simulink model "pro82"  (Simulink 7.4)
settings: Solver=ode45  StartTime=0.0  StopTime=10.0  RelTol=1e-3
undefined symbols (not defined in the file or in its folder): magnitude
libraries: commchan3 x20, commfilt2 x8, dspstat3 x4, dspindex x2, commdigbbndpm3 x2, dspinverses x2, commrandsrc2 x1, commsink2 x1
settings Model: Creator=tjh  LastModifiedBy=tjh

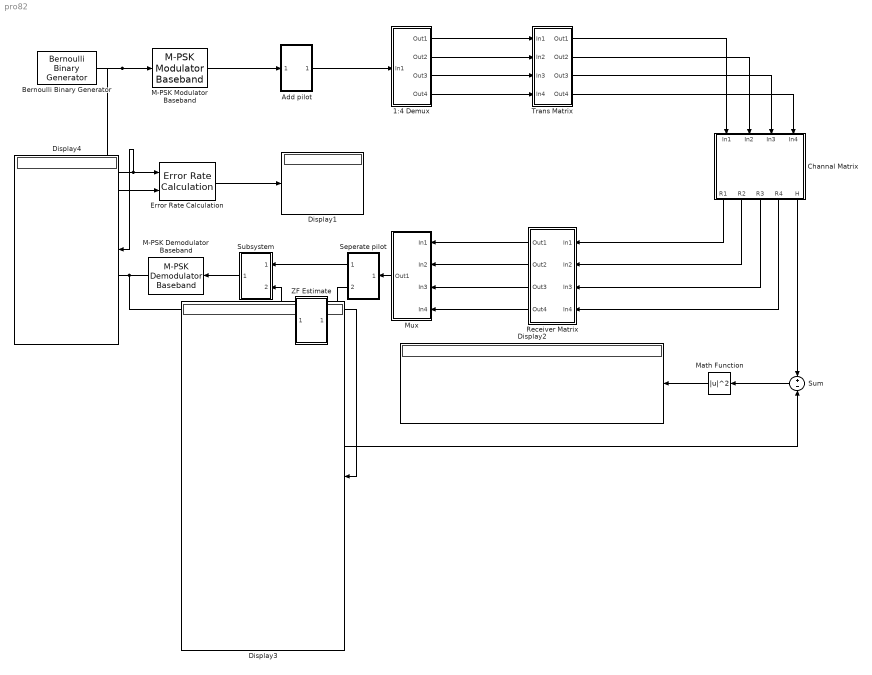
== system pro82 ==
  1:4 Demux : Subsystem
  Add pilot : Subsystem
  Bernoulli Binary Generator : commrandsrc2/Bernoulli Binary Generator  DialogController=commDDGCreate  DialogControllerArgs=DataTag0  SystemSampleTime=-1  P=0.5  seed=61  Ts=1e-4/(4*4*96)  frameBased=on  sampPerFrame=4*4*96  orient=off  outDataType=boolean
  Channal Matrix : Subsystem
  Display{1..4} (4 alike) : Display
  Error Rate Calculation : commsink2/Error Rate Calculation  N=21  st_delay=0  cp_mode=Entire frame  subframe=[]  PMode=Port  WsName=ErrorVec  RsMode2=off  stop=off  numErr=100  maxBits=1e6
  M-PSK Demodulator Baseband : commdigbbndpm3/M-PSK Demodulator Baseband  DialogController=commDDGCreate  DialogControllerArgs=DataTag5  M=16  Ph=pi/16  Dec=Gray  Mapping=[0:7]  OutType=Bit  DecType=Hard decision  VarSource=Dialog  Variance=1  outDtype1=boolean  outDtype2=Inherit via internal rule  derotateFactorWordLen=16
  M-PSK Modulator Baseband : commdigbbndpm3/M-PSK Modulator Baseband  DialogController=commDDGCreate  DialogControllerArgs=DataTag6  M=16  InType=Bit  Enc=Gray  Mapping=[0:7]  Ph=pi/16  outDtype=double  outWordLen=16  outUDDataType=sfix(16)  outFracLenMode=Best precision  outFracLen=15
  Math Function : Math  Operator=magnitude^2  OutDataType=fixdt(1, 16)  OutScaling=2^0  SaturateOnIntegerOverflow=on
  Mux : Subsystem
  Receiver Matrix : Subsystem
  Seperate pilot : Subsystem
  Subsystem : Subsystem
  Sum : Sum  Inputs=+-  OutDataType=fixdt(1, 16)  OutScaling=2^0
  Trans Matrix : Subsystem
  ZF Estimate : Subsystem
  wires:
  Bernoulli Binary Generator/1 -> M-PSK Modulator Baseband/1, Error Rate Calculation/1, Display4/1
  M-PSK Modulator Baseband/1 -> Add pilot/1(In1)
  Add pilot/1(Out1) -> 1:4 Demux/1(In1)
  1:4 Demux/1(Out1) -> Trans Matrix/1(In1)
  1:4 Demux/2(Out2) -> Trans Matrix/2(In2)
  1:4 Demux/3(Out3) -> Trans Matrix/3(In3)
  1:4 Demux/4(Out4) -> Trans Matrix/4(In4)
  Trans Matrix/1(Out1) -> Channal Matrix/1(In1)
  Trans Matrix/3(Out3) -> Channal Matrix/3(In3)
  Channal Matrix/1(R1) -> Receiver Matrix/1(In1)
  Trans Matrix/2(Out2) -> Channal Matrix/2(In2)
  Trans Matrix/4(Out4) -> Channal Matrix/4(In4)
  Channal Matrix/2(R2) -> Receiver Matrix/2(In2)
  Channal Matrix/3(R3) -> Receiver Matrix/3(In3)
  Channal Matrix/4(R4) -> Receiver Matrix/4(In4)
  Receiver Matrix/1(Out1) -> Mux/1(In1)
  Receiver Matrix/2(Out2) -> Mux/2(In2)
  Receiver Matrix/3(Out3) -> Mux/3(In3)
  Receiver Matrix/4(Out4) -> Mux/4(In4)
  Mux/1(Out1) -> Seperate pilot/1(In1)
  Seperate pilot/2(Out2) -> ZF Estimate/1(In1)
  ZF Estimate/1(Out1) -> Subsystem/2(In2), Sum/2
  Seperate pilot/1(Out1) -> Subsystem/1(In1)
  Subsystem/1(Out1) -> M-PSK Demodulator Baseband/1
  M-PSK Demodulator Baseband/1 -> Error Rate Calculation/2, Display3/1
  Error Rate Calculation/1 -> Display1/1
  Channal Matrix/5(H) -> Sum/1
  Sum/1 -> Math Function/1
  Math Function/1 -> Display2/1

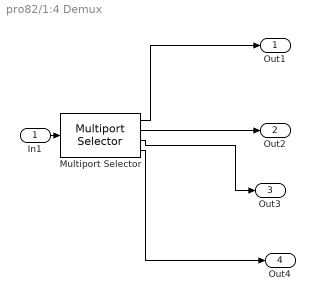
== system pro82/1:4 Demux ==
  In1 : Inport
  Multiport Selector : dspindex/Multiport Selector  rowsOrCols=Rows  idxCellArray={ 1, 2, 3, 4 }  idxErrMode=Clip Index
  Out1 : Outport
  Out2 : Outport  Port=2
  Out3 : Outport  Port=3
  Out4 : Outport  Port=4
  wires:
  Multiport Selector/1 -> Out1/1
  Multiport Selector/2 -> Out2/1
  In1/1 -> Multiport Selector/1
  Multiport Selector/3 -> Out3/1
  Multiport Selector/4 -> Out4/1

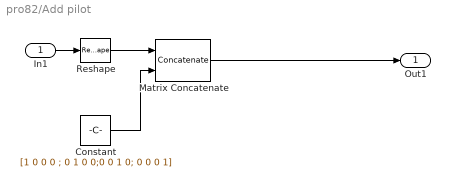
== system pro82/Add pilot ==
  In1 : Inport
  Constant : Constant  Value=[1 0 0 0 ; 0 1 0 0;0 0 1 0; 0 0 0 1]  OutDataType=fixdt(1, 16)  OutScaling=2^0  SampleTime=1e-4
  Matrix Concatenate : Concatenate  Mode=Multidimensional array  ConcatenateDimension=2
  Reshape : Reshape  OutputDimensionality=Customize  OutputDimensions=[4,96]
  Out1 : Outport
  wires:
  Reshape/1 -> Matrix Concatenate/1
  Constant/1 -> Matrix Concatenate/2
  In1/1 -> Reshape/1
  Matrix Concatenate/1 -> Out1/1

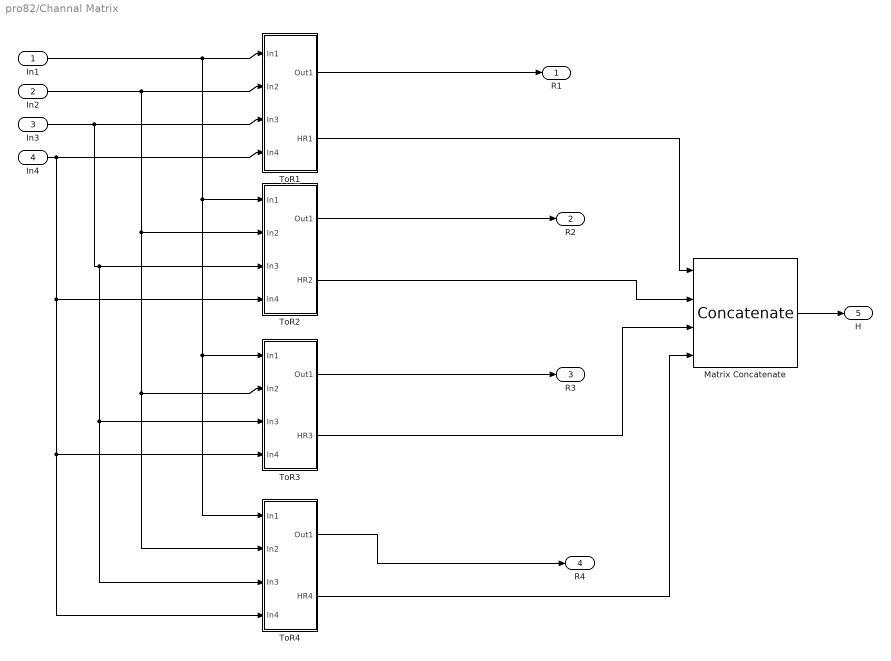
== system pro82/Channal Matrix ==
  In1 : Inport
  In2 : Inport  Port=2
  In3 : Inport  Port=3
  In4 : Inport  Port=4
  Matrix Concatenate : Concatenate  NumInputs=4  Mode=Multidimensional array
  ToR1 : Subsystem
  ToR2 : Subsystem
  ToR3 : Subsystem
  ToR4 : Subsystem
  R1 : Outport
  R2 : Outport  Port=2
  R3 : Outport  Port=3
  R4 : Outport  Port=4
  H : Outport  Port=5
  wires:
  In1/1 -> ToR1/1(In1), ToR2/1(In1), ToR3/1(In1), ToR4/1(In1)
  In2/1 -> ToR1/2(In2), ToR2/2(In2), ToR3/2(In2), ToR4/2(In2)
  ToR1/1(Out1) -> R1/1
  In3/1 -> ToR1/3(In3), ToR2/3(In3), ToR3/3(In3), ToR4/3(In3)
  In4/1 -> ToR1/4(In4), ToR2/4(In4), ToR3/4(In4), ToR4/4(In4)
  ToR2/1(Out1) -> R2/1
  ToR3/1(Out1) -> R3/1
  ToR4/1(Out1) -> R4/1
  ToR1/2(HR1) -> Matrix Concatenate/1
  ToR2/2(HR2) -> Matrix Concatenate/2
  ToR3/2(HR3) -> Matrix Concatenate/3
  ToR4/2(HR4) -> Matrix Concatenate/4
  Matrix Concatenate/1 -> H/1

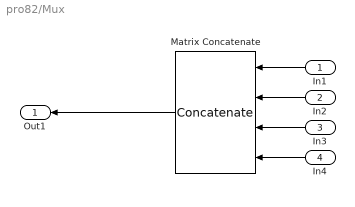
== system pro82/Mux ==
  In1 : Inport
  In2 : Inport  Port=2
  In3 : Inport  Port=3
  In4 : Inport  Port=4
  Matrix Concatenate : Concatenate  NumInputs=4  Mode=Multidimensional array
  Out1 : Outport
  wires:
  In1/1 -> Matrix Concatenate/1
  In2/1 -> Matrix Concatenate/2
  Matrix Concatenate/1 -> Out1/1
  In3/1 -> Matrix Concatenate/3
  In4/1 -> Matrix Concatenate/4

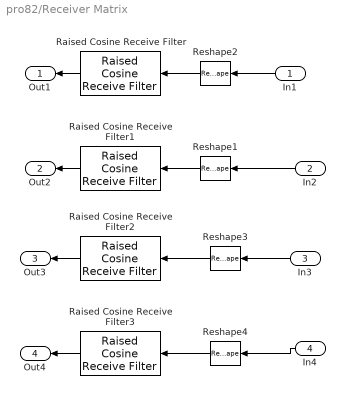
== system pro82/Receiver Matrix ==
  In1 : Inport
  In2 : Inport  Port=2
  In3 : Inport  Port=3
  In4 : Inport  Port=4
  Raised Cosine Receive Filter : commfilt2/Raised Cosine Receive Filter  DialogController=dspDDGCreate  DialogControllerArgs=DataTag7  SystemSampleTime=-1  filtType=Square root  N=8  D=4  R=0.3  sampMode=Mute  saveAsFlag=0  framing=Maintain input frame size  rateMode=Downsampling  downFactor=8  downOffset=0  checkGain=Normalized  filterGain=1  checkCoeff=off  variableName=rcRxFilt  launchFVT=off  roundingMode=Floor  overflowMode=off
  Raised Cosine Receive Filter1 : commfilt2/Raised Cosine Receive Filter  DialogController=dspDDGCreate  DialogControllerArgs=DataTag8  SystemSampleTime=-1  filtType=Square root  N=8  D=4  R=0.3  sampMode=Mute  saveAsFlag=0  framing=Maintain input frame size  rateMode=Downsampling  downFactor=8  downOffset=0  checkGain=Normalized  filterGain=1  checkCoeff=off  variableName=rcRxFilt1  launchFVT=off  roundingMode=Floor  overflowMode=off
  Raised Cosine Receive Filter2 : commfilt2/Raised Cosine Receive Filter  DialogController=dspDDGCreate  DialogControllerArgs=DataTag9  SystemSampleTime=-1  filtType=Square root  N=8  D=4  R=0.3  sampMode=Mute  saveAsFlag=0  framing=Maintain input frame size  rateMode=Downsampling  downFactor=8  downOffset=0  checkGain=Normalized  filterGain=1  checkCoeff=off  variableName=rcRxFilt2  launchFVT=off  roundingMode=Floor  overflowMode=off
  Raised Cosine Receive Filter3 : commfilt2/Raised Cosine Receive Filter  DialogController=dspDDGCreate  DialogControllerArgs=DataTag10  SystemSampleTime=-1  filtType=Square root  N=8  D=4  R=0.3  sampMode=Mute  saveAsFlag=0  framing=Maintain input frame size  rateMode=Downsampling  downFactor=8  downOffset=0  checkGain=Normalized  filterGain=1  checkCoeff=off  variableName=rcRxFilt3  launchFVT=off  roundingMode=Floor  overflowMode=off
  Reshape{1..4} (4 alike) : Reshape  OutputDimensionality=Row vector (2-D)  OutputDimensions=[100,4]
  Out1 : Outport
  Out2 : Outport  Port=2
  Out3 : Outport  Port=3
  Out4 : Outport  Port=4
  wires:
  In1/1 -> Reshape2/1
  In3/1 -> Reshape3/1
  In4/1 -> Reshape4/1
  In2/1 -> Reshape1/1
  Reshape2/1 -> Raised Cosine Receive Filter/1
  Reshape1/1 -> Raised Cosine Receive Filter1/1
  Reshape3/1 -> Raised Cosine Receive Filter2/1
  Reshape4/1 -> Raised Cosine Receive Filter3/1
  Raised Cosine Receive Filter/1 -> Out1/1
  Raised Cosine Receive Filter1/1 -> Out2/1
  Raised Cosine Receive Filter2/1 -> Out3/1
  Raised Cosine Receive Filter3/1 -> Out4/1

== system pro82/Seperate pilot ==
  In1 : Inport
  Multiport Selector : dspindex/Multiport Selector  rowsOrCols=Columns  idxCellArray={[1:96],[97:100]}  idxErrMode=Clip Index
  Out1 : Outport
  Out2 : Outport  Port=2
  wires:
  Multiport Selector/1 -> Out1/1
  Multiport Selector/2 -> Out2/1
  In1/1 -> Multiport Selector/1

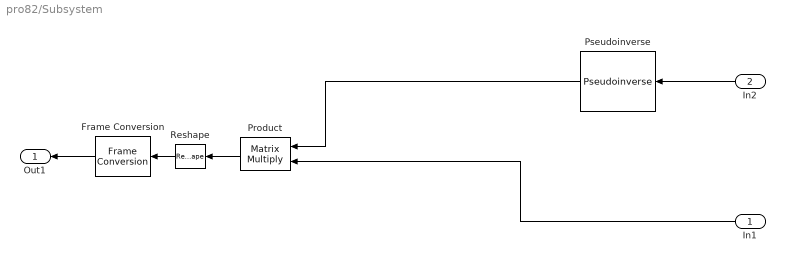
== system pro82/Subsystem ==
  In1 : Inport
  In2 : Inport  Port=2
  Frame Conversion : FrameConversion
  Product : Product  Multiplication=Matrix(*)  OutDataType=fixdt(1, 16)  OutScaling=2^0  RndMeth=Zero
  Pseudoinverse : dspinverses/Pseudoinverse  wanterr=off
  Reshape : Reshape  OutputDimensionality=Column vector (2-D)  OutputDimensions=[4,96]
  Out1 : Outport
  wires:
  Pseudoinverse/1 -> Product/1
  Product/1 -> Reshape/1
  In1/1 -> Product/2
  Reshape/1 -> Frame Conversion/1
  Frame Conversion/1 -> Out1/1
  In2/1 -> Pseudoinverse/1

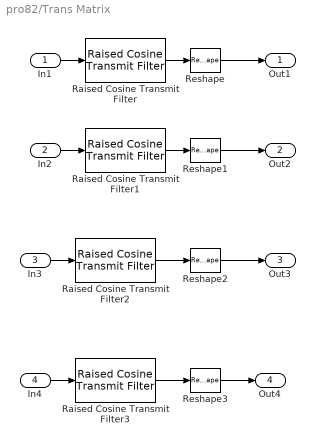
== system pro82/Trans Matrix ==
  In1 : Inport
  In2 : Inport  Port=2
  In3 : Inport  Port=3
  In4 : Inport  Port=4
  Raised Cosine Transmit Filter : commfilt2/Raised Cosine Transmit Filter  DialogController=dspDDGCreate  DialogControllerArgs=DataTag11  SystemSampleTime=-1  filtType=Square root  D=4  R=0.3  sampMode=Mute  saveAsFlag=0  framing=Maintain input frame size  N=8  checkGain=Normalized  filterGain=1  checkCoeff=off  variableName=rcTxFilt  launchFVT=off  roundingMode=Floor  overflowMode=off
  Raised Cosine Transmit Filter1 : commfilt2/Raised Cosine Transmit Filter  DialogController=dspDDGCreate  DialogControllerArgs=DataTag12  SystemSampleTime=-1  filtType=Square root  D=4  R=0.2  sampMode=Mute  saveAsFlag=0  framing=Maintain input frame size  N=8  checkGain=Normalized  filterGain=1  checkCoeff=off  variableName=rcTxFilt1  launchFVT=off  roundingMode=Floor  overflowMode=off
  Raised Cosine Transmit Filter2 : commfilt2/Raised Cosine Transmit Filter  DialogController=dspDDGCreate  DialogControllerArgs=DataTag13  SystemSampleTime=-1  filtType=Square root  D=4  R=0.2  sampMode=Mute  saveAsFlag=0  framing=Maintain input frame size  N=8  checkGain=Normalized  filterGain=1  checkCoeff=off  variableName=rcTxFilt2  launchFVT=off  roundingMode=Floor  overflowMode=off
  Raised Cosine Transmit Filter3 : commfilt2/Raised Cosine Transmit Filter  DialogController=dspDDGCreate  DialogControllerArgs=DataTag14  SystemSampleTime=-1  filtType=Square root  D=4  R=0.2  sampMode=Mute  saveAsFlag=0  framing=Maintain input frame size  N=8  checkGain=Normalized  filterGain=1  checkCoeff=off  variableName=rcTxFilt3  launchFVT=off  roundingMode=Floor  overflowMode=off
  Reshape{,1..3} (4 alike) : Reshape  OutputDimensionality=Column vector (2-D)  OutputDimensions=[100,4]
  Out1 : Outport
  Out2 : Outport  Port=2
  Out3 : Outport  Port=3
  Out4 : Outport  Port=4
  wires:
  In1/1 -> Raised Cosine Transmit Filter/1
  In3/1 -> Raised Cosine Transmit Filter2/1
  In4/1 -> Raised Cosine Transmit Filter3/1
  In2/1 -> Raised Cosine Transmit Filter1/1
  Reshape/1 -> Out1/1
  Reshape1/1 -> Out2/1
  Reshape2/1 -> Out3/1
  Reshape3/1 -> Out4/1
  Raised Cosine Transmit Filter/1 -> Reshape/1
  Raised Cosine Transmit Filter1/1 -> Reshape1/1
  Raised Cosine Transmit Filter2/1 -> Reshape2/1
  Raised Cosine Transmit Filter3/1 -> Reshape3/1

== system pro82/ZF Estimate ==
  In1 : Inport
  Constant : Constant  Value=[1 0 0 0;0 1 0 0;0 0 1 0;0 0 0 1]  OutDataType=fixdt(1, 16)  OutScaling=2^0  SampleTime=1e-4
  Product2 : Product  Multiplication=Matrix(*)  OutDataType=fixdt(1, 16)  OutScaling=2^0  RndMeth=Zero
  Pseudoinverse : dspinverses/Pseudoinverse  wanterr=off
  Out1 : Outport
  wires:
  In1/1 -> Product2/1
  Product2/1 -> Out1/1
  Constant/1 -> Pseudoinverse/1
  Pseudoinverse/1 -> Product2/2

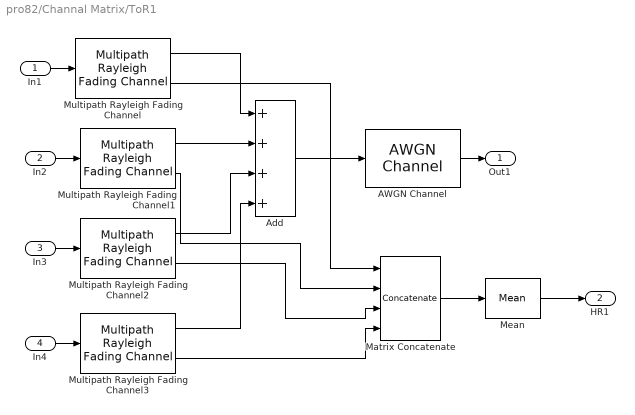
== system pro82/Channal Matrix/ToR1 ==
  In1 : Inport
  In2 : Inport  Port=2
  In3 : Inport  Port=3
  In4 : Inport  Port=4
  AWGN Channel : commchan3/AWGN Channel  SystemSampleTime=-1  seed=73  noiseMode="Signal to noise ratio  (SNR)"  EbNodB=10  EsNodB=10  SNRdB=10  bitsPerSym=4  Ps=0.25/8  Tsym=1e-6  variance=1
  Add : Sum  Inputs=++++  OutDataType=fixdt(1, 16)  OutScaling=2^-10
  Matrix Concatenate : Concatenate  NumInputs=4  Mode=Multidimensional array  ConcatenateDimension=2
  Mean : dspstat3/Mean  DialogController=dspDDGCreate  DialogControllerArgs=DataTag1  run=off  reset_popup=None  directionMode=Each column  dimension=1  treatSBRowAsCol=on  roiEnable=off  roiType=Rectangles  roiPortion=Entire ROI  roiOutput=Individual statistics for each ROI  roiFlag=off  outputDataTypeStr=Inherit: Same as accumulator  outputLastDataTypeStr=Inherit: Same as accumulator  outputMin=[]  outputMax=[]  roundingMode=Floor  overflowMode=off
  Multipath Rayleigh Fading Channel : commchan3/Multipath Rayleigh Fading Channel  SystemSampleTime=-1  maxDopplerShift=40  spectrumType=Jakes  sigmaGaussian=1/sqrt(2)  coeffRounded=[1 -1.72 0.785]  freqMinMaxRJakes=[0 1]  freqMinMaxAJakes=[0 1]  sigmaGaussian1=1/sqrt(2)  sigmaGaussian2=1/sqrt(2)  centerFreqGaussian1=0.0  centerFreqGaussian2=0.0  gainGaussian1=0.5  gainGaussian2=0.5  coeffBell=9  dopplerSpectrum=doppler.jakes  pathDelays=[0]  avgPathGaindB=[0]  normalizePathGains=on  seed=12345  enableProbe=0  openVisAtStart=off  outPathGains=on  outDelay=off
  Multipath Rayleigh Fading Channel1 : commchan3/Multipath Rayleigh Fading Channel  SystemSampleTime=-1  maxDopplerShift=40  spectrumType=Jakes  sigmaGaussian=1/sqrt(2)  coeffRounded=[1 -1.72 0.785]  freqMinMaxRJakes=[0 1]  freqMinMaxAJakes=[0 1]  sigmaGaussian1=1/sqrt(2)  sigmaGaussian2=1/sqrt(2)  centerFreqGaussian1=0.0  centerFreqGaussian2=0.0  gainGaussian1=0.5  gainGaussian2=0.5  coeffBell=9  dopplerSpectrum=doppler.jakes  pathDelays=[0]  avgPathGaindB=[0]  normalizePathGains=on  seed=15678  enableProbe=0  openVisAtStart=off  outPathGains=on  outDelay=off
  Multipath Rayleigh Fading Channel2 : commchan3/Multipath Rayleigh Fading Channel  SystemSampleTime=-1  maxDopplerShift=40  spectrumType=Jakes  sigmaGaussian=1/sqrt(2)  coeffRounded=[1 -1.72 0.785]  freqMinMaxRJakes=[0 1]  freqMinMaxAJakes=[0 1]  sigmaGaussian1=1/sqrt(2)  sigmaGaussian2=1/sqrt(2)  centerFreqGaussian1=0.0  centerFreqGaussian2=0.0  gainGaussian1=0.5  gainGaussian2=0.5  coeffBell=9  dopplerSpectrum=doppler.jakes  pathDelays=[0]  avgPathGaindB=[0]  normalizePathGains=on  seed=13987  enableProbe=0  openVisAtStart=off  outPathGains=on  outDelay=off
  Multipath Rayleigh Fading Channel3 : commchan3/Multipath Rayleigh Fading Channel  SystemSampleTime=-1  maxDopplerShift=40  spectrumType=Jakes  sigmaGaussian=1/sqrt(2)  coeffRounded=[1 -1.72 0.785]  freqMinMaxRJakes=[0 1]  freqMinMaxAJakes=[0 1]  sigmaGaussian1=1/sqrt(2)  sigmaGaussian2=1/sqrt(2)  centerFreqGaussian1=0.0  centerFreqGaussian2=0.0  gainGaussian1=0.5  gainGaussian2=0.5  coeffBell=9  dopplerSpectrum=doppler.jakes  pathDelays=[0]  avgPathGaindB=[0]  normalizePathGains=on  seed=19876  enableProbe=0  openVisAtStart=off  outPathGains=on  outDelay=off
  Out1 : Outport
  HR1 : Outport  Port=2
  wires:
  Multipath Rayleigh Fading Channel/1 -> Add/1
  Multipath Rayleigh Fading Channel1/1 -> Add/2
  Multipath Rayleigh Fading Channel2/1 -> Add/3
  Multipath Rayleigh Fading Channel3/1 -> Add/4
  Add/1 -> AWGN Channel/1
  In1/1 -> Multipath Rayleigh Fading Channel/1
  AWGN Channel/1 -> Out1/1
  In2/1 -> Multipath Rayleigh Fading Channel1/1
  In3/1 -> Multipath Rayleigh Fading Channel2/1
  In4/1 -> Multipath Rayleigh Fading Channel3/1
  Multipath Rayleigh Fading Channel/2 -> Matrix Concatenate/1
  Multipath Rayleigh Fading Channel2/2 -> Matrix Concatenate/3
  Multipath Rayleigh Fading Channel3/2 -> Matrix Concatenate/4
  Matrix Concatenate/1 -> Mean/1
  Multipath Rayleigh Fading Channel1/2 -> Matrix Concatenate/2
  Mean/1 -> HR1/1

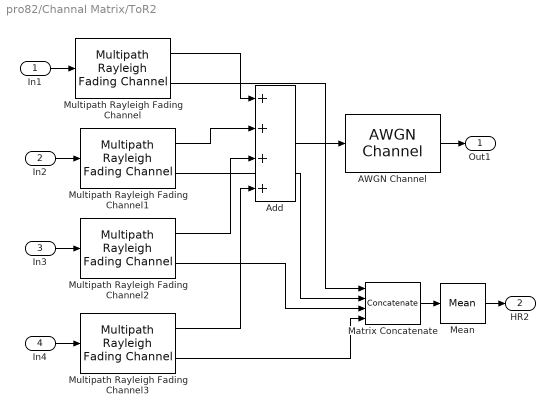
== system pro82/Channal Matrix/ToR2 ==
  In1 : Inport
  In2 : Inport  Port=2
  In3 : Inport  Port=3
  In4 : Inport  Port=4
  AWGN Channel : commchan3/AWGN Channel  SystemSampleTime=-1  seed=210  noiseMode="Signal to noise ratio  (SNR)"  EbNodB=10  EsNodB=10  SNRdB=10  bitsPerSym=4  Ps=0.25/8  Tsym=1e-6  variance=1
  Add : Sum  Inputs=++++  OutDataType=fixdt(1, 16)  OutScaling=2^-10
  Matrix Concatenate : Concatenate  NumInputs=4  Mode=Multidimensional array  ConcatenateDimension=2
  Mean : dspstat3/Mean  DialogController=dspDDGCreate  DialogControllerArgs=DataTag2  run=off  reset_popup=None  directionMode=Each column  dimension=1  treatSBRowAsCol=on  roiEnable=off  roiType=Rectangles  roiPortion=Entire ROI  roiOutput=Individual statistics for each ROI  roiFlag=off  outputDataTypeStr=Inherit: Same as accumulator  outputLastDataTypeStr=Inherit: Same as accumulator  outputMin=[]  outputMax=[]  roundingMode=Floor  overflowMode=off
  Multipath Rayleigh Fading Channel : commchan3/Multipath Rayleigh Fading Channel  SystemSampleTime=-1  maxDopplerShift=40  spectrumType=Jakes  sigmaGaussian=1/sqrt(2)  coeffRounded=[1 -1.72 0.785]  freqMinMaxRJakes=[0 1]  freqMinMaxAJakes=[0 1]  sigmaGaussian1=1/sqrt(2)  sigmaGaussian2=1/sqrt(2)  centerFreqGaussian1=0.0  centerFreqGaussian2=0.0  gainGaussian1=0.5  gainGaussian2=0.5  coeffBell=9  dopplerSpectrum=doppler.jakes  pathDelays=[0]  avgPathGaindB=[0]  normalizePathGains=on  seed=2  enableProbe=0  openVisAtStart=off  outPathGains=on  outDelay=off
  Multipath Rayleigh Fading Channel1 : commchan3/Multipath Rayleigh Fading Channel  SystemSampleTime=-1  maxDopplerShift=40  spectrumType=Jakes  sigmaGaussian=1/sqrt(2)  coeffRounded=[1 -1.72 0.785]  freqMinMaxRJakes=[0 1]  freqMinMaxAJakes=[0 1]  sigmaGaussian1=1/sqrt(2)  sigmaGaussian2=1/sqrt(2)  centerFreqGaussian1=0.0  centerFreqGaussian2=0.0  gainGaussian1=0.5  gainGaussian2=0.5  coeffBell=9  dopplerSpectrum=doppler.jakes  pathDelays=[0]  avgPathGaindB=[0]  normalizePathGains=on  seed=23456  enableProbe=0  openVisAtStart=off  outPathGains=on  outDelay=off
  Multipath Rayleigh Fading Channel2 : commchan3/Multipath Rayleigh Fading Channel  SystemSampleTime=-1  maxDopplerShift=40  spectrumType=Jakes  sigmaGaussian=1/sqrt(2)  coeffRounded=[1 -1.72 0.785]  freqMinMaxRJakes=[0 1]  freqMinMaxAJakes=[0 1]  sigmaGaussian1=1/sqrt(2)  sigmaGaussian2=1/sqrt(2)  centerFreqGaussian1=0.0  centerFreqGaussian2=0.0  gainGaussian1=0.5  gainGaussian2=0.5  coeffBell=9  dopplerSpectrum=doppler.jakes  pathDelays=[0]  avgPathGaindB=[0]  normalizePathGains=on  seed=29876  enableProbe=0  openVisAtStart=off  outPathGains=on  outDelay=off
  Multipath Rayleigh Fading Channel3 : commchan3/Multipath Rayleigh Fading Channel  SystemSampleTime=-1  maxDopplerShift=40  spectrumType=Jakes  sigmaGaussian=1/sqrt(2)  coeffRounded=[1 -1.72 0.785]  freqMinMaxRJakes=[0 1]  freqMinMaxAJakes=[0 1]  sigmaGaussian1=1/sqrt(2)  sigmaGaussian2=1/sqrt(2)  centerFreqGaussian1=0.0  centerFreqGaussian2=0.0  gainGaussian1=0.5  gainGaussian2=0.5  coeffBell=9  dopplerSpectrum=doppler.jakes  pathDelays=[0]  avgPathGaindB=[0]  normalizePathGains=on  seed=27345  enableProbe=0  openVisAtStart=off  outPathGains=on  outDelay=off
  Out1 : Outport
  HR2 : Outport  Port=2
  wires:
  In4/1 -> Multipath Rayleigh Fading Channel3/1
  In3/1 -> Multipath Rayleigh Fading Channel2/1
  In2/1 -> Multipath Rayleigh Fading Channel1/1
  AWGN Channel/1 -> Out1/1
  In1/1 -> Multipath Rayleigh Fading Channel/1
  Add/1 -> AWGN Channel/1
  Multipath Rayleigh Fading Channel3/1 -> Add/4
  Multipath Rayleigh Fading Channel2/1 -> Add/3
  Multipath Rayleigh Fading Channel1/1 -> Add/2
  Multipath Rayleigh Fading Channel/1 -> Add/1
  Multipath Rayleigh Fading Channel/2 -> Matrix Concatenate/1
  Multipath Rayleigh Fading Channel1/2 -> Matrix Concatenate/2
  Multipath Rayleigh Fading Channel2/2 -> Matrix Concatenate/3
  Multipath Rayleigh Fading Channel3/2 -> Matrix Concatenate/4
  Matrix Concatenate/1 -> Mean/1
  Mean/1 -> HR2/1

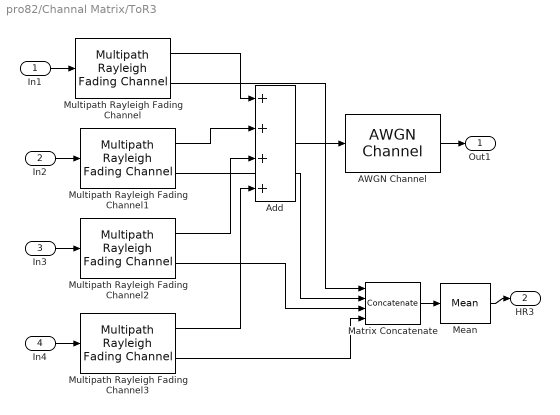
== system pro82/Channal Matrix/ToR3 ==
  In1 : Inport
  In2 : Inport  Port=2
  In3 : Inport  Port=3
  In4 : Inport  Port=4
  AWGN Channel : commchan3/AWGN Channel  SystemSampleTime=-1  seed=310  noiseMode="Signal to noise ratio  (SNR)"  EbNodB=10  EsNodB=10  SNRdB=10  bitsPerSym=4  Ps=0.25/8  Tsym=1e-6  variance=1
  Add : Sum  Inputs=++++  OutDataType=fixdt(1, 16)  OutScaling=2^-10
  Matrix Concatenate : Concatenate  NumInputs=4  Mode=Multidimensional array  ConcatenateDimension=2
  Mean : dspstat3/Mean  DialogController=dspDDGCreate  DialogControllerArgs=DataTag3  run=off  reset_popup=None  directionMode=Each column  dimension=1  treatSBRowAsCol=on  roiEnable=off  roiType=Rectangles  roiPortion=Entire ROI  roiOutput=Individual statistics for each ROI  roiFlag=off  outputDataTypeStr=Inherit: Same as accumulator  outputLastDataTypeStr=Inherit: Same as accumulator  outputMin=[]  outputMax=[]  roundingMode=Floor  overflowMode=off
  Multipath Rayleigh Fading Channel : commchan3/Multipath Rayleigh Fading Channel  SystemSampleTime=-1  maxDopplerShift=40  spectrumType=Jakes  sigmaGaussian=1/sqrt(2)  coeffRounded=[1 -1.72 0.785]  freqMinMaxRJakes=[0 1]  freqMinMaxAJakes=[0 1]  sigmaGaussian1=1/sqrt(2)  sigmaGaussian2=1/sqrt(2)  centerFreqGaussian1=0.0  centerFreqGaussian2=0.0  gainGaussian1=0.5  gainGaussian2=0.5  coeffBell=9  dopplerSpectrum=doppler.jakes  pathDelays=[0]  avgPathGaindB=[0]  normalizePathGains=on  seed=34567  enableProbe=0  openVisAtStart=off  outPathGains=on  outDelay=off
  Multipath Rayleigh Fading Channel1 : commchan3/Multipath Rayleigh Fading Channel  SystemSampleTime=-1  maxDopplerShift=40  spectrumType=Jakes  sigmaGaussian=1/sqrt(2)  coeffRounded=[1 -1.72 0.785]  freqMinMaxRJakes=[0 1]  freqMinMaxAJakes=[0 1]  sigmaGaussian1=1/sqrt(2)  sigmaGaussian2=1/sqrt(2)  centerFreqGaussian1=0.0  centerFreqGaussian2=0.0  gainGaussian1=0.5  gainGaussian2=0.5  coeffBell=9  dopplerSpectrum=doppler.jakes  pathDelays=[0]  avgPathGaindB=[0]  normalizePathGains=on  seed=39876  enableProbe=0  openVisAtStart=off  outPathGains=on  outDelay=off
  Multipath Rayleigh Fading Channel2 : commchan3/Multipath Rayleigh Fading Channel  SystemSampleTime=-1  maxDopplerShift=40  spectrumType=Jakes  sigmaGaussian=1/sqrt(2)  coeffRounded=[1 -1.72 0.785]  freqMinMaxRJakes=[0 1]  freqMinMaxAJakes=[0 1]  sigmaGaussian1=1/sqrt(2)  sigmaGaussian2=1/sqrt(2)  centerFreqGaussian1=0.0  centerFreqGaussian2=0.0  gainGaussian1=0.5  gainGaussian2=0.5  coeffBell=9  dopplerSpectrum=doppler.jakes  pathDelays=[0]  avgPathGaindB=[0]  normalizePathGains=on  seed=36512  enableProbe=0  openVisAtStart=off  outPathGains=on  outDelay=off
  Multipath Rayleigh Fading Channel3 : commchan3/Multipath Rayleigh Fading Channel  SystemSampleTime=-1  maxDopplerShift=40  spectrumType=Jakes  sigmaGaussian=1/sqrt(2)  coeffRounded=[1 -1.72 0.785]  freqMinMaxRJakes=[0 1]  freqMinMaxAJakes=[0 1]  sigmaGaussian1=1/sqrt(2)  sigmaGaussian2=1/sqrt(2)  centerFreqGaussian1=0.0  centerFreqGaussian2=0.0  gainGaussian1=0.5  gainGaussian2=0.5  coeffBell=9  dopplerSpectrum=doppler.jakes  pathDelays=[0]  avgPathGaindB=[0]  normalizePathGains=on  seed=31111  enableProbe=0  openVisAtStart=off  outPathGains=on  outDelay=off
  Out1 : Outport
  HR3 : Outport  Port=2
  wires:
  Matrix Concatenate/1 -> Mean/1
  Multipath Rayleigh Fading Channel3/2 -> Matrix Concatenate/4
  Multipath Rayleigh Fading Channel2/2 -> Matrix Concatenate/3
  Multipath Rayleigh Fading Channel1/2 -> Matrix Concatenate/2
  Multipath Rayleigh Fading Channel/2 -> Matrix Concatenate/1
  Multipath Rayleigh Fading Channel/1 -> Add/1
  Multipath Rayleigh Fading Channel1/1 -> Add/2
  Multipath Rayleigh Fading Channel2/1 -> Add/3
  Multipath Rayleigh Fading Channel3/1 -> Add/4
  Add/1 -> AWGN Channel/1
  In1/1 -> Multipath Rayleigh Fading Channel/1
  AWGN Channel/1 -> Out1/1
  In2/1 -> Multipath Rayleigh Fading Channel1/1
  In3/1 -> Multipath Rayleigh Fading Channel2/1
  In4/1 -> Multipath Rayleigh Fading Channel3/1
  Mean/1 -> HR3/1

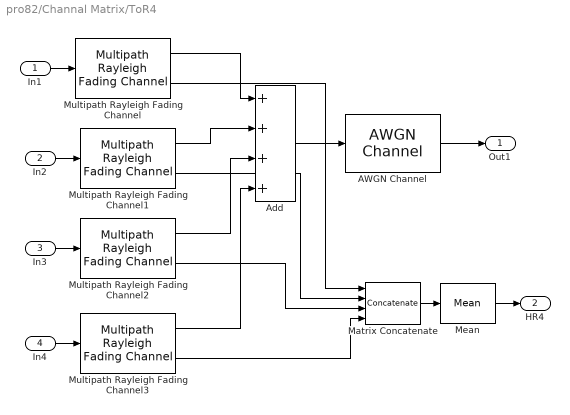
== system pro82/Channal Matrix/ToR4 ==
  In1 : Inport
  In2 : Inport  Port=2
  In3 : Inport  Port=3
  In4 : Inport  Port=4
  AWGN Channel : commchan3/AWGN Channel  SystemSampleTime=-1  seed=310  noiseMode="Signal to noise ratio  (SNR)"  EbNodB=10  EsNodB=10  SNRdB=10  bitsPerSym=4  Ps=0.25/8  Tsym=1e-6  variance=1
  Add : Sum  Inputs=++++  OutDataType=fixdt(1, 16)  OutScaling=2^-10
  Matrix Concatenate : Concatenate  NumInputs=4  Mode=Multidimensional array  ConcatenateDimension=2
  Mean : dspstat3/Mean  DialogController=dspDDGCreate  DialogControllerArgs=DataTag4  run=off  reset_popup=None  directionMode=Each column  dimension=1  treatSBRowAsCol=on  roiEnable=off  roiType=Rectangles  roiPortion=Entire ROI  roiOutput=Individual statistics for each ROI  roiFlag=off  outputDataTypeStr=Inherit: Same as accumulator  outputLastDataTypeStr=Inherit: Same as accumulator  outputMin=[]  outputMax=[]  roundingMode=Floor  overflowMode=off
  Multipath Rayleigh Fading Channel : commchan3/Multipath Rayleigh Fading Channel  SystemSampleTime=-1  maxDopplerShift=40  spectrumType=Jakes  sigmaGaussian=1/sqrt(2)  coeffRounded=[1 -1.72 0.785]  freqMinMaxRJakes=[0 1]  freqMinMaxAJakes=[0 1]  sigmaGaussian1=1/sqrt(2)  sigmaGaussian2=1/sqrt(2)  centerFreqGaussian1=0.0  centerFreqGaussian2=0.0  gainGaussian1=0.5  gainGaussian2=0.5  coeffBell=9  dopplerSpectrum=doppler.jakes  pathDelays=[0]  avgPathGaindB=[0]  normalizePathGains=on  seed=55555  enableProbe=0  openVisAtStart=off  outPathGains=on  outDelay=off
  Multipath Rayleigh Fading Channel1 : commchan3/Multipath Rayleigh Fading Channel  SystemSampleTime=-1  maxDopplerShift=40  spectrumType=Jakes  sigmaGaussian=1/sqrt(2)  coeffRounded=[1 -1.72 0.785]  freqMinMaxRJakes=[0 1]  freqMinMaxAJakes=[0 1]  sigmaGaussian1=1/sqrt(2)  sigmaGaussian2=1/sqrt(2)  centerFreqGaussian1=0.0  centerFreqGaussian2=0.0  gainGaussian1=0.5  gainGaussian2=0.5  coeffBell=9  dopplerSpectrum=doppler.jakes  pathDelays=[0]  avgPathGaindB=[0]  normalizePathGains=on  seed=66666  enableProbe=0  openVisAtStart=off  outPathGains=on  outDelay=off
  Multipath Rayleigh Fading Channel2 : commchan3/Multipath Rayleigh Fading Channel  SystemSampleTime=-1  maxDopplerShift=40  spectrumType=Jakes  sigmaGaussian=1/sqrt(2)  coeffRounded=[1 -1.72 0.785]  freqMinMaxRJakes=[0 1]  freqMinMaxAJakes=[0 1]  sigmaGaussian1=1/sqrt(2)  sigmaGaussian2=1/sqrt(2)  centerFreqGaussian1=0.0  centerFreqGaussian2=0.0  gainGaussian1=0.5  gainGaussian2=0.5  coeffBell=9  dopplerSpectrum=doppler.jakes  pathDelays=[0]  avgPathGaindB=[0]  normalizePathGains=on  seed=77777  enableProbe=0  openVisAtStart=off  outPathGains=on  outDelay=off
  Multipath Rayleigh Fading Channel3 : commchan3/Multipath Rayleigh Fading Channel  SystemSampleTime=-1  maxDopplerShift=40  spectrumType=Jakes  sigmaGaussian=1/sqrt(2)  coeffRounded=[1 -1.72 0.785]  freqMinMaxRJakes=[0 1]  freqMinMaxAJakes=[0 1]  sigmaGaussian1=1/sqrt(2)  sigmaGaussian2=1/sqrt(2)  centerFreqGaussian1=0.0  centerFreqGaussian2=0.0  gainGaussian1=0.5  gainGaussian2=0.5  coeffBell=9  dopplerSpectrum=doppler.jakes  pathDelays=[0]  avgPathGaindB=[0]  normalizePathGains=on  seed=88888  enableProbe=0  openVisAtStart=off  outPathGains=on  outDelay=off
  Out1 : Outport
  HR4 : Outport  Port=2
  wires:
  In4/1 -> Multipath Rayleigh Fading Channel3/1
  In3/1 -> Multipath Rayleigh Fading Channel2/1
  In2/1 -> Multipath Rayleigh Fading Channel1/1
  AWGN Channel/1 -> Out1/1
  In1/1 -> Multipath Rayleigh Fading Channel/1
  Add/1 -> AWGN Channel/1
  Multipath Rayleigh Fading Channel3/1 -> Add/4
  Multipath Rayleigh Fading Channel2/1 -> Add/3
  Multipath Rayleigh Fading Channel1/1 -> Add/2
  Multipath Rayleigh Fading Channel/1 -> Add/1
  Multipath Rayleigh Fading Channel/2 -> Matrix Concatenate/1
  Multipath Rayleigh Fading Channel1/2 -> Matrix Concatenate/2
  Multipath Rayleigh Fading Channel2/2 -> Matrix Concatenate/3
  Multipath Rayleigh Fading Channel3/2 -> Matrix Concatenate/4
  Matrix Concatenate/1 -> Mean/1
  Mean/1 -> HR4/1
